simulink subsystem "nplib_state"  (R2024b)
settings: Solver=VariableStepAuto  StartTime=0.0  StopTime=10.0  RelTol=1e-3
undefined symbols (not defined in the file): Earth, F, init, Light, MIL, terrain, WGS84, wind, WMM2020
libraries: aerolibasang x5, aerolibwind2 x3, aerolibtransform2 x2, aerolibatmos2 x1, aerolibgravity2 x1
settings Model: Creator=CETCA  LastModifiedBy=CETCA

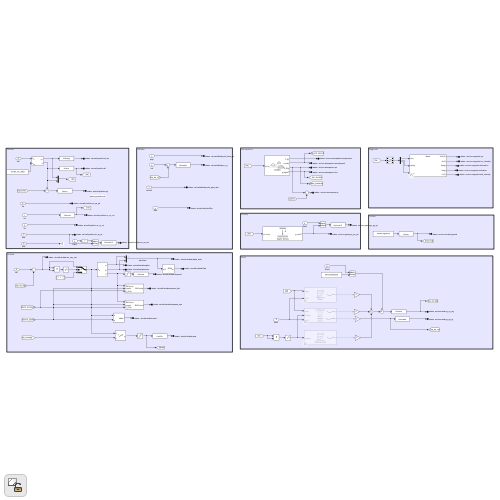
[thumbnail: Simulink's stored preview of the top-level diagram]
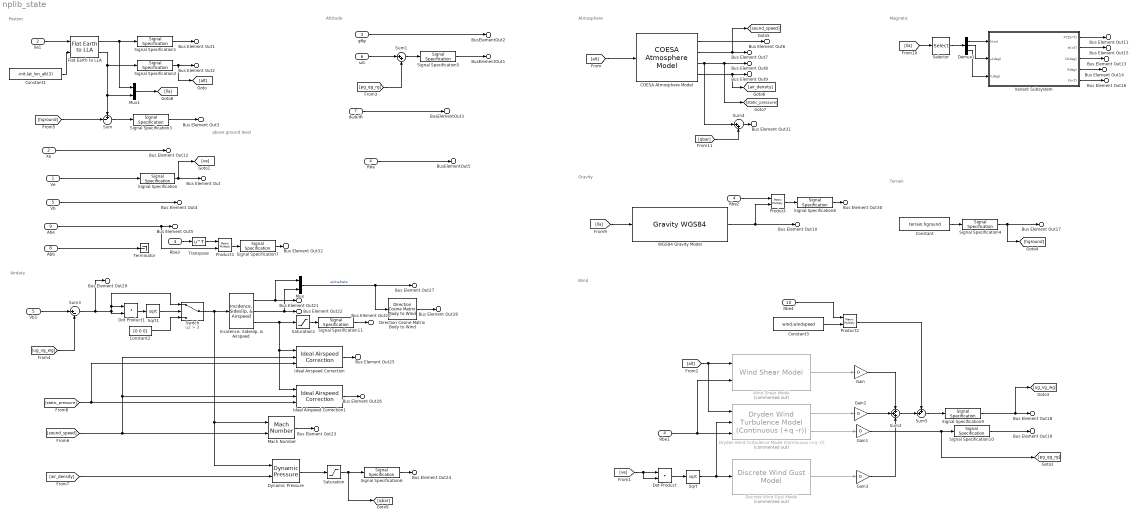
== system nplib_state ==
  note: above ground level
  note: Postion
  note: Attitude
  note: Atmosphere
  note: Gravity
  note: Magnetic
  note: Terrain
  note: Wind
  note: Airdata
  Ve : Inport
  Xe : Inport  Port=2
  φθψ : Inport  Port=3
  Rbe : Inport  Port=4
  Vb : Inport  Port=5
  ωb : Inport  Port=6
  dωb/dt : Inport  Port=7
  Abb : Inport  Port=8
  Abe : Inport  Port=9
  Rbe4 : Inport  Port=10
  COESA Atmosphere Model : aerolibatmos2/COESA Atmosphere Model  units=Metric (MKS)  spec=1976 COESA-extended U.S. Standard Atmosphere  model=Profile  profile_var=High temperature  profile_percent=1%  profile_alt=5 km (16404 ft)  envelope_var=High temperature  envelope_percent=1%  action=Warning
  Constant : Constant  Value=terrain.hground
  Constant1 : Constant  Value=-init.lat_lon_alt(3)
  Constant2 : Constant  Value=[0 0 0]
  Constant3 : Constant  Value=wind.windspeed
  Demux1 : Demux  Outputs=3
  Direction Cosine Matrix Body to Wind : aerolibtransform2/Direction Cosine Matrix Body to Wind
  Discrete Wind Gust Model : aerolibwind2/Discrete Wind Gust Model  Commented=on  units=Metric (MKS)  Gx=on  Gy=on  Gz=on  t_0=5  d_m=[120 120 80]  v_m=[3.5 3.5 3.0]
  Dot Product : DotProduct  OutDataTypeStr=Inherit: Inherit via internal rule
  Dot Product1 : DotProduct  OutDataTypeStr=Inherit: Inherit via internal rule
  Dryden Wind Turbulence Model (Continuous (+q -r)) : aerolibwind2/Dryden Wind Turbulence Model  (Continuous (+q -r))  Commented=on  units=Metric (MKS)  spec=MIL-F-8785C  model=Continuous Dryden (+q -r)  W20=15  Wdeg=0  TurbProb=10^-2 - Light  L_high=533.4  Wingspan=10  ts=0.1  Seed=[23341 23342 23343 23344]  T_on=on
  Dynamic Pressure : aerolibasang/Dynamic Pressure
  Flat Earth to LLA : aerolibtransform2/Flat Earth to LLA  units=Metric (MKS)  ptype=Earth (WGS84)  F=1/298.257223563  R=6378137  refPosPort=off  LL0=init.lat_lon_alt(1:2)  psi=0
  Gain{,1..3} (4 alike) : Gain  Gain=0
  Ideal Airspeed Correction : aerolibasang/Ideal Airspeed Correction  units=Metric (MKS)  vel_in=TAS  vel_out_tas=CAS  vel_out_eas=TAS  vel_out_cas=TAS  method=Table Lookup  SubOnly=off  action=None
  Ideal Airspeed Correction1 : aerolibasang/Ideal Airspeed Correction  units=Metric (MKS)  vel_in=TAS  vel_out_tas=EAS  vel_out_eas=TAS  vel_out_cas=TAS  method=Table Lookup  SubOnly=off  action=None
  "Incidence, Sideslip, & Airspeed" : aerolibasang/Incidence, Sideslip, & Airspeed
  Mach Number : aerolibasang/Mach Number
  Mux : Mux  Inputs=2
  Mux1 : Mux  Inputs=2
  Product : Product  Multiplication=Matrix(*)
  Product1 : Product  Multiplication=Matrix(*)
  Product2 : Product  Multiplication=Matrix(*)
  Rbe1 : InportShadow  Port=4
  Rbe2 : InportShadow  Port=4
  Rbe3 : InportShadow  Port=4
  Saturation : Saturate  UpperLimit=inf  LowerLimit=eps
  Saturation1 : Saturate  UpperLimit=inf  LowerLimit=eps
  Selector : Selector  InputPortWidth=3  IndexOptions=Index vector (dialog)  Indices=[3 1 2]  OutputSizes=1
  Signal Specification : SignalSpecification  Unit=m/s
  Signal Specification1 : SignalSpecification  Unit=deg
  Signal Specification10 : SignalSpecification  Unit=rad/s
  Signal Specification11 : SignalSpecification  Unit=m/s
  Signal Specification2 : SignalSpecification  Unit=m
  Signal Specification3 : SignalSpecification  Unit=m
  Signal Specification4 : SignalSpecification  Unit=m
  Signal Specification5 : SignalSpecification  Unit=rad/s
  Signal Specification6 : SignalSpecification  Unit=Pa
  Signal Specification7 : SignalSpecification  Unit=m/s^2
  Signal Specification8 : SignalSpecification  Unit=m/s^2
  Signal Specification9 : SignalSpecification  Unit=m/s
  Sqrt : Sqrt
  Sqrt1 : Sqrt
  Sum : Sum  Inputs=+-|
  Sum1 : Sum  Inputs=|++
  Sum2 : Sum  Inputs=+++
  Sum3 : Sum  Inputs=|+-
  Sum4 : Sum  Inputs=|++
  Sum5 : Sum  Inputs=++|
  Switch : Switch  Criteria=u2 > Threshold  Threshold=3  SaturateOnIntegerOverflow=off  InputSameDT=off
  Terminator : Terminator
  Transpose : Math  Operator=transpose
  Variant Subsystem : Subsystem  Variant=on
  Vb1 : InportShadow  Port=5
  "WGS84 Gravity Model  " : GravityWGS84
  Wind Shear Model : aerolibwind2/Wind Shear Model  Commented=on  units=Metric (MKS)  phase=Category C - Terminal Flight Phase  W_20=15  Wdeg=0
  Xe1 : InportShadow  Port=2
  Bus Element Out1 : Outport  PortName=states  Element=aircraft.position.lat_lon
  Bus Element Out2 : Outport  PortName=states  Element=aircraft.position.alt
  Bus Element Out3 : Outport  PortName=states  Element=aircraft.position.agl
  Bus Element Out12 : Outport  PortName=states  Element=aircraft.position.pn_pe_pd
  Bus Element Out : Outport  PortName=states  Element=aircraft.position.vn_ve_vd
  Bus Element Out4 : Outport  PortName=states  Element=aircraft.position.vx_vy_vz
  Bus Element Out32 : Outport  PortName=states  Element=aircraft.position.an_ae_ad
  Bus Element Out5 : Outport  PortName=states  Element=aircraft.position.ax_ay_az
  BusElementOut2 : Outport  PortName=states  Element=aircraft.attitude.phi_theta_psi
  BusElementOut1 : Outport  PortName=states  Element=aircraft.attitude.p_q_r
  BusElementOut3 : Outport  PortName=states  Element=aircraft.attitude.pdot_qdot_rdot
  BusElementOut5 : Outport  PortName=states  Element=aircraft.attitude.Rbe
  Bus Element Out20 : Outport  PortName=states  Element=aircraft.airdata.airspeed
  Bus Element Out21 : Outport  PortName=states  Element=aircraft.airdata.alpha
  Bus Element Out22 : Outport  PortName=states  Element=aircraft.airdata.beta
  Bus Element Out23 : Outport  PortName=states  Element=aircraft.airdata.mach
  Bus Element Out24 : Outport  PortName=states  Element=aircraft.airdata.qbar
  Bus Element Out25 : Outport  PortName=states  Element=aircraft.airdata.airspeed_cali
  Bus Element Out26 : Outport  PortName=states  Element=aircraft.airdata.airspeed_equ
  Bus Element Out27 : Outport  PortName=states  Element=aircraft.airdata.alpha_beta
  Bus Element Out28 : Outport  PortName=states  Element=aircraft.airdata.Rwb
  Bus Element Out29 : Outport  PortName=states  Element=aircraft.airdata.vax_vay_vaz
  Bus Element Out6 : Outport  PortName=states  Element=environ.atmosphere.temperature
  Bus Element Out7 : Outport  PortName=states  Element=environ.atmosphere.soundspeed
  Bus Element Out8 : Outport  PortName=states  Element=environ.atmosphere.ps
  Bus Element Out9 : Outport  PortName=states  Element=environ.atmosphere.rho
  Bus Element Out31 : Outport  PortName=states  Element=environ.atmosphere.pt
  Bus Element Out10 : Outport  PortName=states  Element=environ.gravity.gn_ge_gd
  Bus Element Out30 : Outport  PortName=states  Element=environ.gravity.gx_gy_gz
  Bus Element Out11 : Outport  PortName=states  Element=environ.magnetic.xyz
  Bus Element Out13 : Outport  PortName=states  Element=environ.magnetic.declination
  Bus Element Out14 : Outport  PortName=states  Element=environ.magnetic.inclination
  Bus Element Out15 : Outport  PortName=states  Element=environ.magnetic.hor_intensity
  Bus Element Out16 : Outport  PortName=states  Element=environ.magnetic.total_intensity
  Bus Element Out17 : Outport  PortName=states  Element=environ.terrain.hground
  Bus Element Out18 : Outport  PortName=states  Element=environ.wind.ug_vg_wg
  Bus Element Out19 : Outport  PortName=states  Element=environ.wind.pg_qg_rg
  wires:
  Signal Specification6/1 -> Bus Element Out24/1
  Signal Specification5/1 -> BusElementOut1/1
  Gain3/1 -> Sum2/3
  Gain2/1 -> Sum2/2
  Gain/1 -> Sum2/1
  Mux/1 -> Bus Element Out27/1, Direction Cosine Matrix Body to Wind/1  "alpha/beta"
  Ideal Airspeed Correction1/1 -> Bus Element Out26/1
  Ideal Airspeed Correction/1 -> Bus Element Out25/1
  [static_pressure] -> Ideal Airspeed Correction/3, Ideal Airspeed Correction1/3
  [air_density] -> Dynamic Pressure/2
  Mach Number/1 -> Bus Element Out23/1
  [sound_speed] -> Mach Number/2, Ideal Airspeed Correction1/2, Ideal Airspeed Correction/2
  "Incidence, Sideslip, & Airspeed"/1 -> Mux/1, Bus Element Out21/1
  "Incidence, Sideslip, & Airspeed"/2 -> Mux/2, Bus Element Out22/1
  "Incidence, Sideslip, & Airspeed"/3 -> Ideal Airspeed Correction/1, Ideal Airspeed Correction1/1, Saturation1/1
  Sum3/1 -> Bus Element Out29/1, Dot Product1/2, Dot Product1/1, Switch/1
  [ug_vg_wg] -> Sum3/2
  Vb1/1 -> Sum3/1
  Gain1/1 -> [pg_qg_rg], Signal Specification10/1
  Wind Shear Model/1 -> Gain/1
  Sqrt/1 -> Dryden Wind Turbulence Model (Continuous (+q -r))/2, Discrete Wind Gust Model/1
  Dot Product/1 -> Sqrt/1
  [ve] -> Dot Product/2, Dot Product/1
  [alt] -> Wind Shear Model/1, Dryden Wind Turbulence Model (Continuous (+q -r))/1
  Rbe1/1 -> Wind Shear Model/2, Dryden Wind Turbulence Model (Continuous (+q -r))/3
  Dryden Wind Turbulence Model (Continuous (+q -r))/2 -> Gain1/1
  Discrete Wind Gust Model/1 -> Gain3/1
  Dryden Wind Turbulence Model (Continuous (+q -r))/1 -> Gain2/1
  Signal Specification4/1 -> [hground], Bus Element Out17/1
  Constant/1 -> Signal Specification4/1
  Variant Subsystem/5(F(nT)) -> Bus Element Out16/1
  Variant Subsystem/2(H(nT)) -> Bus Element Out15/1
  Variant Subsystem/4(I(deg)) -> Bus Element Out14/1
  Variant Subsystem/3(D(deg)) -> Bus Element Out13/1
  Demux1/3 -> Variant Subsystem/3(l(deg))
  Demux1/2 -> Variant Subsystem/2(μ(deg))
  Demux1/1 -> Variant Subsystem/1(h(m))
  Selector/1 -> Demux1/1
  [lla] -> Selector/1
  "WGS84 Gravity Model  "/1 -> Bus Element Out10/1, Product/2
  [lla] -> "WGS84 Gravity Model  "/1
  COESA Atmosphere Model/4 -> [air_density], Bus Element Out9/1
  COESA Atmosphere Model/3 -> [static_pressure], Bus Element Out8/1, Sum4/1
  COESA Atmosphere Model/2 -> [sound_speed], Bus Element Out7/1
  COESA Atmosphere Model/1 -> Bus Element Out6/1
  [alt] -> COESA Atmosphere Model/1
  Xe/1 -> Bus Element Out12/1
  dωb/dt/1 -> BusElementOut3/1
  [pg_qg_rg] -> Sum1/2
  Sum1/1 -> Signal Specification5/1
  ωb/1 -> Sum1/1
  Rbe/1 -> BusElementOut5/1
  φθψ/1 -> BusElementOut2/1
  Abe/1 -> Bus Element Out5/1, Product1/2
  Vb/1 -> Bus Element Out4/1
  [hground] -> Sum/2
  Signal Specification3/1 -> Bus Element Out3/1
  Sum/1 -> Signal Specification3/1
  Signal Specification2/1 -> [alt], Bus Element Out2/1
  Signal Specification1/1 -> Bus Element Out1/1
  Signal Specification/1 -> [ve], Bus Element Out/1
  Ve/1 -> Signal Specification/1
  Xe1/1 -> Flat Earth to LLA/1
  Flat Earth to LLA/1 -> Signal Specification1/1, Mux1/1
  Flat Earth to LLA/2 -> Signal Specification2/1, Mux1/2, Sum/1
  Constant1/1 -> Flat Earth to LLA/2
  Mux1/1 -> [lla]
  Variant Subsystem/1(XYZ(nT)) -> Bus Element Out11/1
  Direction Cosine Matrix Body to Wind/1 -> Bus Element Out28/1
  Dot Product1/1 -> Sqrt1/1
  Sqrt1/1 -> Switch/2
  Constant2/1 -> Switch/3
  Switch/1 -> "Incidence, Sideslip, & Airspeed"/1, Dynamic Pressure/1, Mach Number/1
  Dynamic Pressure/1 -> Saturation/1
  Saturation/1 -> Signal Specification6/1, [qbar]
  Saturation1/1 -> Signal Specification11/1
  Rbe2/1 -> Product/1
  Product/1 -> Signal Specification8/1
  Abb/1 -> Terminator/1
  Sum4/1 -> Bus Element Out31/1
  [qbar] -> Sum4/2
  Sum2/1 -> Sum5/2
  Sum5/1 -> Signal Specification9/1
  Rbe3/1 -> Transpose/1
  Product1/1 -> Signal Specification7/1
  Transpose/1 -> Product1/1
  Signal Specification7/1 -> Bus Element Out32/1
  Signal Specification8/1 -> Bus Element Out30/1
  Signal Specification9/1 -> Bus Element Out18/1, [ug_vg_wg]
  Signal Specification10/1 -> Bus Element Out19/1
  Signal Specification11/1 -> Bus Element Out20/1
  Rbe4/1 -> Product2/1
  Constant3/1 -> Product2/2
  Product2/1 -> Sum5/1

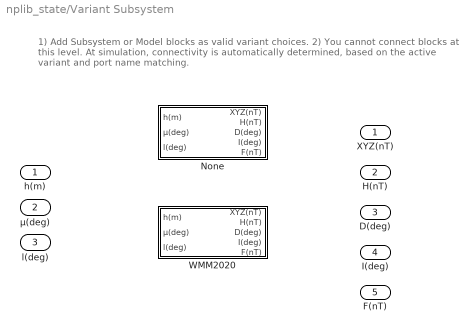
== system nplib_state/Variant Subsystem ==
  note: 1) Add Subsystem or Model blocks as valid variant choices.
      | 2) You cannot connect blocks at this level. At simulation, connectivity is automatically
      | determined, based on the active variant and port name matching.
  h(m) : Inport
  μ(deg) : Inport  Port=2
  l(deg) : Inport  Port=3
  None : Subsystem  VariantControl=true
  WMM2020 : Subsystem  VariantControl=false
  XYZ(nT) : Outport
  H(nT) : Outport  Port=2
  D(deg) : Outport  Port=3
  I(deg) : Outport  Port=4
  F(nT) : Outport  Port=5

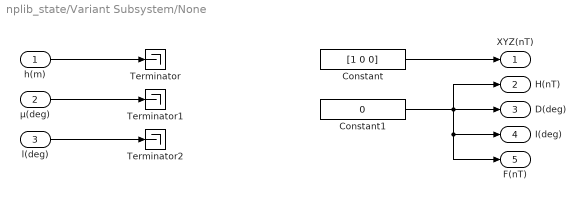
== system nplib_state/Variant Subsystem/None ==
  h(m) : Inport
  μ(deg) : Inport  Port=2
  l(deg) : Inport  Port=3
  Constant : Constant  Value=[1 0 0]
  Constant1 : Constant  Value=0
  Terminator : Terminator
  Terminator1 : Terminator
  Terminator2 : Terminator
  XYZ(nT) : Outport
  H(nT) : Outport  Port=2
  D(deg) : Outport  Port=3
  I(deg) : Outport  Port=4
  F(nT) : Outport  Port=5
  wires:
  Constant1/1 -> D(deg)/1, H(nT)/1, I(deg)/1, F(nT)/1
  Constant/1 -> XYZ(nT)/1
  μ(deg)/1 -> Terminator1/1
  l(deg)/1 -> Terminator2/1
  h(m)/1 -> Terminator/1

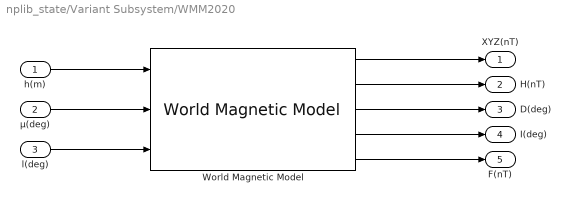
== system nplib_state/Variant Subsystem/WMM2020 ==
  h(m) : Inport
  μ(deg) : Inport  Port=2
  l(deg) : Inport  Port=3
  World Magnetic Model : aerolibgravity2/World Magnetic Model  model=WMM2020 (2020-2025)  customFile='WMM2020.COF'  units=Metric (MKS)  time_in=off  month=January  day=1  year=2020  action=Error  h_out=on  dec_out=on  inc_out=on  ti_out=on
  XYZ(nT) : Outport
  H(nT) : Outport  Port=2
  D(deg) : Outport  Port=3
  I(deg) : Outport  Port=4
  F(nT) : Outport  Port=5
  wires:
  μ(deg)/1 -> World Magnetic Model/2
  l(deg)/1 -> World Magnetic Model/3
  World Magnetic Model/5 -> F(nT)/1
  World Magnetic Model/4 -> I(deg)/1
  World Magnetic Model/3 -> D(deg)/1
  World Magnetic Model/2 -> H(nT)/1
  World Magnetic Model/1 -> XYZ(nT)/1
  h(m)/1 -> World Magnetic Model/1
